simulink library "sm_car_4post_lib"  (R2021b)
settings: Solver=VariableStepAuto  StartTime=0.0  StopTime=10.0  RelTol=1e-3
values from neighbouring files (symbols this model uses):
  Init = struct    [sm_car_4post_init_data.m]
  N = 100    [sm_extr_data_cam_roller_curve.m]
  s = sin(q)    [sm_extr_data_cam_roller_curve.m]
  Vehicle = Vehicle_03    [sm_car_4post_gen_op.m]    (also in sm_car_4post_testrig_plot2testall.m)
undefined symbols (not defined in the file or in its folder): clr_upr, hp_in_f_ua, hp_in_r_ua, hp_la_out, hp_ua_out, LAc, LAf, LAr, opc_upr, radius_upr, rhs_hp, sm_car_4post_platform, smcar_param, UAc, UAf, UAr, X, Y, Z
libraries: sm_lib x234, $bdroot x71, fl_lib x24, nesl_utility x21, simulink x3
(part 1 of 11)
Description:
  | Simscape Vehicle Templates Library
settings Model: Creator=The MathWorks, Inc.  LastModifiedBy=The MathWorks, Inc.
settings SolverCC: AlgebraicLoopSolver=TrustRegion
settings DataIOCC: ReturnWorkspaceOutputs=off
settings DebuggingCC: PregeneratedLibrarySubsystemCodeDiagnostic=none  SFMachineParentedDataDiag=warning  ArithmeticOperatorsInVariantConditions=warning
settings SFSimCC: SimUseLocalCustomCode=off  CustomCodeUndefinedFunction=UseInterfaceOnly
settings RTWCC: RTWUseLocalCustomCode=off

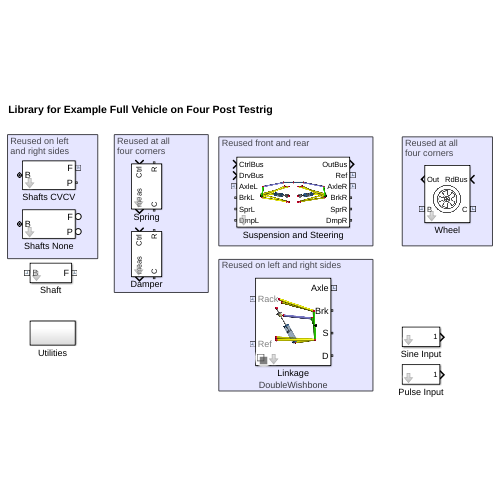
[thumbnail: Simulink's stored preview of the top-level diagram]
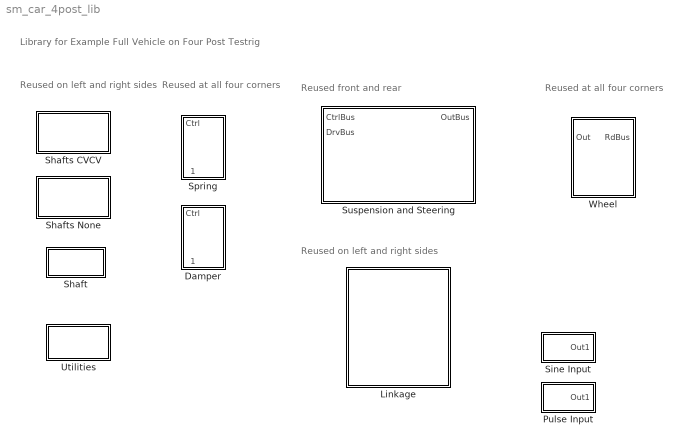
== system sm_car_4post_lib ==
  note: Reused at all
      | four corners
  note: Reused on left and right sides
  note: Reused front and rear
  note: Reused on left
      | and right sides
  note: Library for Example Full Vehicle on Four Post Testrig
  note: Reused at all
      | four corners
  Damper : Subsystem  mask(Damper){Damper=Vehicle.Chassis.Damper.Rear}
      mask prompts: Damper "Damper Parameters"
  Linkage : Subsystem  Variant=on  VariantControlMode=label  VariantControl=Variant1  LabelModeActiveChoice=DoubleWishbone  mask(Suspension){popup_leftRight=Right, Linkage=Vehicle.Chassis.SuspF.Linkage, Init=Init, VariantLabel=Vehicle.Chassis.SuspF.Linkage.class.Value, InitTriggerDropdown=1}
      mask prompts: popup_leftRight "Left/Right"; Linkage "Linkage Parameters"; Init "Initial Values"; VariantLabel "Variant Label"; InitTriggerDropdown "Initialization Trigger Dropdown"
      mask help: Suspension with multiple variants. Variants are configured by parameter Variant Label. Parameter values are contained within Linkage Parameters.
      mask init:
      | curblk = gcb;
      | 
      | % Set variant for this block 
      | set_param(curblk,'LabelModeActiveChoice',VariantLabel);
      | 
      | % Trigger Mask Initialization for 
      | % variant subsystems below this level
      | sm_car_4post_lib_maskInitTrigger(curblk)
      | 
      | % Set Left/Right fields
      | 
      | sm_car_4post_lib_setLeftRight(curblk,'variant');
      settings: AttributesFormatString=%<ActiveVariant>
      mask TypeOptions popup_leftRight: Left | Right
      mask TypeOptions InitTriggerDropdown: 0 | 1
      mask Display: image(fullfile(matlabroot,'toolbox','physmod','sm','smdemos','car_4post_testrig','images','sm_car_4post_dwbR_IMAGE.png'));
  Pulse Input : Subsystem  mask(Smooth Pulse){rise_time=0.1, pulse_length=2, wave_amplitude=5, wave_delay=1}
      mask prompts: rise_time "Rise/Fall Time (sec)"; pulse_length "Pulse Length (sec)"; wave_amplitude "Amplitude (m)"; wave_delay "Delay (sec)"
      mask help: Produces a pulse with a smooth start and finish, starting at a chosen time.
  Shaft : Subsystem  mask(Shaft){popup_leftRight=Left, shaft_m=3.5, len_shaft=0.4, clr_shaft=smcar_param.gray, opc_shaft=smcar_param.part.opc, rad_shaft=0.025}
      mask prompts: popup_leftRight "Left/Right"; shaft_m "Shaft Mass (kg)"; len_shaft "Shaft Length (m)"; clr_shaft "Color [RGB]"; opc_shaft "Opacity (0-1)"; rad_shaft "Radius (m)"
      mask help: Rigid shaft model with basic parameterization.
      mask init:
      | if(popup_leftRight == 1)
      |     rhs_shaft = 1;
      | elseif(popup_leftRight == 2)
      |     rhs_shaft = -1;
      | end
      mask TypeOptions popup_leftRight: Left | Right
      mask TypeOptions shaft_m: Shaft/Mass
      mask TypeOptions clr_shaft: Shaft/GraphicDiffuseColor
      mask TypeOptions opc_shaft: Shaft/GraphicOpacity
      mask TypeOptions rad_shaft: Shaft/CylinderRadius
      mask DialogControl cont_vis_shaft Prompt: Visualization
  Shafts CVCV : Subsystem  mask(Driveshafts){popup_leftRight=Right, Shaft=Vehicle.Driveline.ShaftsFL}
      mask prompts: popup_leftRight "Left/Right"; Shaft "Shaft Parameters"
      mask help: Driveshafts from differential to axle.
      mask init:
      | sm_car_4post_lib_setLeftRight(gcb, 'variant');
      mask TypeOptions popup_leftRight: Left | Right
  Shafts None : Subsystem  mask(Driveshaft Open Connection){popup_leftRight=Left, Shaft=Vehicle.Driveline.ShaftsRL}
      mask prompts: popup_leftRight "Left/Right"; Shaft "Shaft Parameters"
      mask help: Variant with no shaft connections, intended as a simple variant or placeholder.
      mask init:
      | sm_car_4post_lib_setLeftRight(gcb, 'variant');
      mask TypeOptions popup_leftRight: Left | Right
  Sine Input : Subsystem  mask(Sine Wave){wave_period=2, num_periods=2, wave_amplitude=5, wave_delay=1}
      mask prompts: wave_period "Period (sec)"; num_periods "Number of cycles"; wave_amplitude "Amplitude (m)"; wave_delay "Delay (sec)"
      mask help: Produces a fixed number of sine waves at a single amplitude and period, starting at a chosen time.
  Spring : Subsystem  mask(Spring){Spring=Vehicle.Chassis.Spring.Front}
      mask prompts: Spring "Spring Parameters"
  Suspension and Steering : Subsystem  mask(Suspension and Steering){Susp=Vehicle.Chassis.SuspF, Init=Init.Front, InitTriggerDropdown=0}
      mask prompts: Susp "Suspension Parameters"; Init "Initial Values"; InitTriggerDropdown "Initialization Trigger Dropdown"
      mask help: Suspension and steering system for front or rear axle.
      mask init:
      | curblk = gcb;
      | % Trigger Mask Initialization for 
      | % variant subsystems below this level
      | sm_car_4post_lib_maskInitTrigger(curblk)
      mask TypeOptions InitTriggerDropdown: 0 | 1
      mask Display: image(fullfile(matlabroot,'toolbox','physmod','sm','smdemos','car_4post_testrig','images','sm_car_4post_suspf_IMAGE.png'));
  Utilities : Subsystem
  Wheel : Subsystem  mask{popup_leftRight=Left, Tire=Vehicle.Chassis.TyreF}
      mask prompts: popup_leftRight "Left/Right"; Tire "Tire Parameters"
      mask init:
      | sm_car_4post_lib_setLeftRight(gcb,'variant');
      mask TypeOptions popup_leftRight: Left | Right
      mask Display: image(fullfile(matlabroot,'toolbox','physmod','sm','smdemos','car_4post_testrig','images','sm_car_4post_wheel_IMAGE.png'));

== system sm_car_4post_lib/Damper ==
  Ctrl : Inport
  Linear : Subsystem  VariantControl=Linear  mask(Linear Damper with Hard Stop){dam_b=Damper.Damping.d.Value, hp_dpr_top=Damper.Damping.sTop.Value, hp_dpr_bot=Damper.Damping.sBottom.Value, bs_lim_upper=Damper.Endstop.xMax.Value, bs_lim_lower=Damper.Endstop.xMin.Value, bs_k_upper=Damper.Endstop.KxMax.Value, bs_k_lower=Damper.Endstop.KxMin.Value, bs_b_upper=Damper.Endstop.dxMax.Value, bs_b_lower=Damper.Endstop.dxMin.Value, bs_region=Damper.Endstop.xTransition.Value}
      mask prompts: dam_b "Damper (N/(m/s))"; hp_dpr_top "HP Damper Top [xyz] (m)"; hp_dpr_bot "HP Damper Bottom [xyz] (m)"; bs_region "Transition Region (m)"
      mask help: Damper and hard stop with linear behavior with measurements.
      mask init:
      | dam_x0 = norm(hp_dpr_top - hp_dpr_bot);
      mask TypeOptions dam_b: Damper/D
      mask DialogControl text_bumpstop_upper Prompt: Upper
      mask DialogControl text_bumpstop_lower Prompt: Lower
      mask DialogControl text_bumpstop_limit Prompt: Limit (m)
      mask DialogControl text_bumpstop_k Prompt: Stiffness (N/m)
      mask DialogControl text_bumpstop_b Prompt: Damping  (N/(m/s))
  R : PMIOPort  Side=Left
  C : PMIOPort  Port=2  Side=Right
  meas : Outport  VectorParamsAs1DForOutWhenUnconnected=off
  wires:
  Linear/1(meas) -> meas/1
  Ctrl/1 -> Linear/1(Ctrl)
  connections:
  Linear/LConn1 -- R/RConn1
  Linear/RConn1 -- C/RConn1

== system sm_car_4post_lib/Linkage ==
  DoubleWishbone : Subsystem  VariantControl=DoubleWishbone  mask(Double-Wishbone Suspension){popup_leftRight=Right, hp_in_f_ua=Linkage.UpperWishbone.sInboardF.Value, hp_in_r_ua=Linkage.UpperWishbone.sInboardR.Value, hp_out_ua=Linkage.UpperWishbone.sOutboard.Value, hp_in_f_la=Linkage.LowerWishbone.sInboardF.Value, hp_in_r_la=Linkage.LowerWishbone.sInboardR.Value, hp_out_la=Linkage.LowerWishbone.sOutboard.Value, hp_upr_cg=Linkage.Upright.sCG.Value, hp_upr_wc=Linkage.Upright.sWheelCentre.Value, hp_in_rod=Linkage.TrackRod.sInboard.Value, hp_upr_rod=Linkage.TrackRod.sOutboard.Value, hp_spr_top=Linkage.Shock.sTop.Value, hp_spr_bot=Linkage.Shock.sBottom.Value, clr_hp=smcar_param.hp.clr, opc_hp=smcar_param.hp.opc, size_hp=0.025, ua_mass=Linkage.UpperWishbone.m.Value, clr_ua=smcar_param.yellow, opc_ua=smcar_param.part.opc, radius_ua=0.02, la_mass=Linkage.LowerWishbone.m.Value, clr_la=smcar_param.yellow, opc_la=smcar_param.part.opc, radius_la=0.02, shock_pist_mass=Linkage.Shock.mPiston.Value, shock_cyl_mass=Linkage.Shock.mCylinder.Value, up_lim_bumpstop=Linkage.Endstop.xMax.Value, low_lim_bumpstop=Linkage.Endstop.xMin.Value, clr_conn_shock=smcar_param.hp.clr, opc_conn_shock=smcar_param.hp.opc, size_conn_shock=0.025, clr_shock_cyl=smcar_param.blue, opc_shock_cyl=1.0, radius_shock_cyl=0.05, clr_shock_piston=smcar_param.gray, opc_shock_piston=1.0, clr_shock_bumpstop=smcar_param.yellowpale, opc_shock_bumpstop=1.0, deadvol_len_shock_cyl=smcar_param.shock.dead_length, piston_len_shock=smcar_param.shock.piston, cyl_cap_len_shock=smcar_param.shock.cap, bumpstop_len_shock=smcar_param.shock.bumpstop_len, upr_mass=Linkage.Upright.m.Value, atoe=Linkage.Upright.aToe.Value, acamber=Linkage.Upright.aCamber.Value, clr_conn_upr=smcar_param.hp.clr, opc_conn_upr=smcar_param.hp.opc, size_conn_upr=smcar_param.hp.rad, clr_upr=smcar_param.green, opc_upr=smcar_param.part.opc, radius_upr=0.02, clr_stub_axle=smcar_param.black, opc_stub_axle=smcar_param.part.opc, radius_stub_axle=0.02, rod_mass=Linkage.TrackRod.m.Value, clr_conn_rod=smcar_param.hp.clr, opc_conn_rod=smcar_param.hp.opc, size_conn_rod=smcar_param.hp.rad, clr_rod=smcar_param.purple, opc_rod=smcar_param.part.opc, radius_rod=0.02, whl_init_spd_lr=Init.nWheel.Value, whlind=1}
      mask prompts: popup_leftRight "Left/Right"; hp_in_f_ua "Upper Arm Front [xyz] (m)"; hp_in_r_ua "Upper Arm Rear [xyz] (m)"; hp_out_ua "Upper Arm Outboard [xyz] (m)"; hp_in_f_la "Lower Arm Front [xyz] (m)"; hp_in_r_la "Lower Arm Rear [xyz] (m)"; hp_out_la "Lower Arm Outboard [xyz] (m)"; hp_upr_cg "Upright CG [xyz] (m)"; hp_upr_wc "Wheel Center [xyz] (m)"; hp_in_rod "Track Rod Inboard [xyz] (m)"; hp_upr_rod "Track Rod Outboard [xyz] (m)"; hp_spr_top "Spring Top [xyz] (m)"; hp_spr_bot "Spring Bottom [xyz] (m)"; ua_mass "Mass (kg)"; clr_ua "Color [RGB]"; opc_ua "Opacity (0-1)"; radius_ua "Radius (m)"; la_mass "Mass (kg)"; clr_la "Color [RGB]"; opc_la "Opacity (0-1)"; radius_la "Radius (m)"; shock_pist_mass "Piston Mass (kg)"; shock_cyl_mass "Cylinder Mass (kg)"; up_lim_bumpstop "Upper Limit (m)"; low_lim_bumpstop "Lower Limit (m)"; deadvol_len_shock_cyl "Dead Volume Height (m)"; piston_len_shock "Piston Length (m)"; cyl_cap_len_shock "Cylinder Cap Length (m)"; bumpstop_len_shock "Bumpstop Length (m)"; upr_mass "Mass (kg)"; atoe "Toe Angle (deg)"; acamber "Camber Angle (deg)"; rod_mass "Mass (kg)"; whl_init_spd_lr "Initial Wheel Speed (rad/s)"; whlind "Wheel Index"
      mask help: This models a double-wishbone suspension for steered and non-steered configurations. The non-steered configuration maintains its orientation via the track rods that connect to fixed points on the subframe.
      mask init:
      | sm_car_4post_lib_setLeftRight(gcb,'none');
      | 
      | if(popup_leftRight == 1)
      |     rhs_susp = 1;
      |     whlind = 1;
      | elseif(popup_leftRight == 2)
      |     rhs_susp = -1;
      |     whlind = 2;
      | end
      mask TypeOptions popup_leftRight: Left | Right
      mask TypeOptions hp_in_f_ua: Upper Arm/hp_in_f | Hardpoints/hp_in_f_ua
      mask TypeOptions hp_in_r_ua: Upper Arm/hp_in_r | Hardpoints/hp_in_r_ua
      mask TypeOptions hp_out_ua: Upper Arm/hp_out | Upright/hp_ua_out
      mask TypeOptions hp_in_f_la: Lower Arm/hp_in_f | Hardpoints/hp_in_f_la
      mask TypeOptions hp_in_r_la: Lower Arm/hp_in_r | Hardpoints/hp_in_r_la
      mask TypeOptions hp_out_la: Lower Arm/hp_out | Upright/hp_la_out
      mask TypeOptions hp_upr_cg: Upright/hp_upr_cg
      mask TypeOptions hp_upr_wc: Upright/hp_upr_wc
      mask TypeOptions hp_in_rod: Track Rod/hp_in
      mask TypeOptions hp_upr_rod: Track Rod/hp_out | Upright/hp_upr_rod
      mask TypeOptions hp_spr_top: Hardpoints/hp_spr_top | Shock/hp_spr_top
      mask TypeOptions hp_spr_bot: Lower Arm/hp_spr | Shock/hp_spr_bot
      mask TypeOptions clr_hp: Hardpoints/clr_hp
      mask TypeOptions opc_hp: Hardpoints/opc_hp
      mask TypeOptions size_hp: Hardpoints/size_hp
      mask TypeOptions ua_mass: Upper Arm/ua_mass
      mask TypeOptions clr_ua: Upper Arm/clr_ua
      mask TypeOptions opc_ua: Upper Arm/opc_ua
      mask TypeOptions radius_ua: Upper Arm/radius_ua
      mask TypeOptions la_mass: Lower Arm/la_mass
      mask TypeOptions clr_la: Lower Arm/clr_la
      mask TypeOptions opc_la: Lower Arm/opc_la
      mask TypeOptions radius_la: Lower Arm/radius_la
      mask TypeOptions shock_pist_mass: Shock/shock_pist_mass
      mask TypeOptions shock_cyl_mass: Shock/shock_cyl_mass
      mask TypeOptions up_lim_bumpstop: Shock/up_lim_bumpstop
      mask TypeOptions low_lim_bumpstop: Shock/low_lim_bumpstop
      mask TypeOptions clr_conn_shock: Shock/clr_conn_shock
      mask TypeOptions opc_conn_shock: Shock/opc_conn_shock
      mask TypeOptions size_conn_shock: Shock/size_conn_shock
      mask TypeOptions clr_shock_cyl: Shock/clr_shock_cyl
      mask TypeOptions opc_shock_cyl: Shock/opc_shock_cyl
      mask TypeOptions radius_shock_cyl: Shock/radius_shock_cyl
      mask TypeOptions clr_shock_piston: Shock/clr_shock_piston
      mask TypeOptions opc_shock_piston: Shock/opc_shock_piston
      mask TypeOptions clr_shock_bumpstop: Shock/clr_shock_bumpstop
      mask TypeOptions opc_shock_bumpstop: Shock/opc_shock_bumpstop
      mask TypeOptions deadvol_len_shock_cyl: Shock/deadvol_len_shock_cyl
      mask TypeOptions piston_len_shock: Shock/piston_len_shock
      mask TypeOptions cyl_cap_len_shock: Shock/cyl_cap_len_shock
      mask TypeOptions bumpstop_len_shock: Shock/bumpstop_len_shock
      mask TypeOptions upr_mass: Upright/upr_mass
      mask TypeOptions atoe: Upright/atoe
      mask TypeOptions acamber: Upright/acamber
      mask TypeOptions clr_conn_upr: Upright/clr_conn_upr
      mask TypeOptions opc_conn_upr: Upright/opc_conn_upr
      mask TypeOptions size_conn_upr: Upright/size_conn_upr
      mask TypeOptions clr_upr: Upright/clr_upr
      mask TypeOptions opc_upr: Upright/opc_upr
      mask TypeOptions radius_upr: Upright/radius_upr
      mask TypeOptions clr_stub_axle: Upright/clr_stub_axle
      mask TypeOptions opc_stub_axle: Upright/opc_stub_axle
      mask TypeOptions radius_stub_axle: Upright/radius_stub_axle
      mask TypeOptions rod_mass: Track Rod/rod_mass
      mask TypeOptions clr_conn_rod: Track Rod/clr_conn_rod
      mask TypeOptions opc_conn_rod: Track Rod/opc_conn_rod
      mask TypeOptions size_conn_rod: Track Rod/size_conn_rod
      mask TypeOptions clr_rod: Track Rod/clr_rod
      mask TypeOptions opc_rod: Track Rod/opc_rod
      mask TypeOptions radius_rod: Track Rod/radius_rod
      mask DialogControl cont_hp Prompt: Hardpoints
      mask DialogControl cont_vis_hp Prompt: Visualization
      mask DialogControl text_clr_hp Prompt: Color [RGB]
      mask DialogControl text_opc_hp Prompt: Opac. (0-1)
      mask DialogControl text_size_hp Prompt: Size (m)
      mask DialogControl text_hp Prompt: Hardpoints
      mask DialogControl cont_ua Prompt: UA
      mask DialogControl cont_vis_ua Prompt: Visualization
      mask DialogControl cont_la Prompt: LA
      mask DialogControl cont_vis_la Prompt: Visualization
      mask DialogControl cont_shock Prompt: Shock
      mask DialogControl cont_parts Prompt: Parts
      mask DialogControl cont_bumpstop Prompt: Bumpstop
      mask DialogControl cont_vis_shock Prompt: Visualization
      mask DialogControl text_clr_shock Prompt: Color  [RGB]
      mask DialogControl text_opc_shock Prompt: Opac. (0-1)
      mask DialogControl text_size_shock Prompt: Size (m)
      mask DialogControl text_conn_shock Prompt: Connections
      mask DialogControl text_shock_shock Prompt: Cylinder
      mask DialogControl text_shock_piston Prompt: Piston
      mask DialogControl text_piston_radius Prompt: <cylinder radius>
      mask DialogControl text_shock_bumpstop Prompt: Bumpstop
      mask DialogControl text_bumpstop_radius Prompt: <cylinder radius>
      mask DialogControl cont_upright Prompt: Upright
      mask DialogControl grp_upright Prompt: Upright
      mask DialogControl cont_vis_upr Prompt: Visualization
      mask DialogControl text_clr_upr Prompt: Color [RGB]
      mask DialogControl text_opc_upr Prompt: Opac. (0-1)
      mask DialogControl text_size_upr Prompt: Size (m)
      mask DialogControl text_conn_upr Prompt: Connections
      mask DialogControl text_upright Prompt: Upright
      mask DialogControl text_stub_axle Prompt: Stub Axle
      mask DialogControl cont_steer Prompt: Steer
      mask DialogControl grp_rod Prompt: Rod
      mask DialogControl cont_vis_rod Prompt: Visualization
      mask DialogControl text_clr_rod Prompt: Color [RGB]
      mask DialogControl text_opc_rod Prompt: Opac. (0-1)
      mask DialogControl text_size_rod Prompt: Size (m)
      mask DialogControl text_conn_rod Prompt: Connections
      mask DialogControl text_rod_rod Prompt: Rod
      mask DialogControl cont_init Prompt: Initial
      mask Display: image(fullfile(matlabroot,'toolbox','physmod','sm','smdemos','car_4post_testrig','images','sm_car_4post_dwbR_IMAGE.png'));
  FiveLinkShockRear : Subsystem  VariantControl=FiveLinkShockRear  mask(Five-Link Suspension, Shock to Rear){popup_leftRight=Right, hp_in_f_ua=Linkage.UpperArmF.sInboard.Value, hp_in_r_ua=Linkage.UpperArmR.sInboard.Value, hp_out_f_ua=Linkage.UpperArmF.sOutboard.Value, hp_out_r_ua=Linkage.UpperArmR.sOutboard.Value, hp_in_f_la=Linkage.LowerArmF.sInboard.Value, hp_in_r_la=Linkage.LowerArmR.sInboard.Value, hp_out_f_la=Linkage.LowerArmF.sOutboard.Value, hp_out_r_la=Linkage.LowerArmR.sOutboard.Value, hp_upr_cg=Linkage.Upright.sCG.Value, hp_upr_wc=Linkage.Upright.sWheelCentre.Value, hp_in_rod=Linkage.TrackRod.sInboard.Value, hp_upr_rod=Linkage.TrackRod.sOutboard.Value, hp_spr_top=Linkage.Shock.sTop.Value, hp_spr_bot=Linkage.Shock.sBottom.Value, clr_hp=smcar_param.hp.clr, opc_hp=smcar_param.hp.opc, size_hp=0.025, uaf_mass=Linkage.UpperArmF.m.Value, uar_mass=Linkage.UpperArmR.m.Value, laf_mass=Linkage.LowerArmF.m.Value, lar_mass=Linkage.LowerArmR.m.Value, clr_conn_links=smcar_param.hp.clr, opc_conn_links=smcar_param.hp.opc, size_conn_links=smcar_param.hp.rad, clr_uaf=smcar_param.yellow, opc_uaf=smcar_param.part.opc, radius_uaf=0.02, clr_uar=smcar_param.yellow, opc_uar=smcar_param.part.opc, radius_uar=0.02, clr_laf=smcar_param.yellow, opc_laf=smcar_param.part.opc, radius_laf=0.02, clr_lar=smcar_param.yellow, opc_lar=smcar_param.part.opc, radius_lar=0.02, shock_pist_mass=Linkage.Shock.mPiston.Value, shock_cyl_mass=Linkage.Shock.mCylinder.Value, up_lim_bumpstop=Linkage.Endstop.xMax.Value, low_lim_bumpstop=Linkage.Endstop.xMin.Value, clr_conn_shock=smcar_param.hp.clr, opc_conn_shock=smcar_param.hp.opc, size_conn_shock=0.025, clr_shock_cyl=smcar_param.blue, opc_shock_cyl=1.0, radius_shock_cyl=0.05, clr_shock_piston=smcar_param.gray, opc_shock_piston=1.0, clr_shock_bumpstop=smcar_param.yellowpale, opc_shock_bumpstop=1.0, deadvol_len_shock_cyl=smcar_param.shock.dead_length, piston_len_shock=smcar_param.shock.piston, cyl_cap_len_shock=smcar_param.shock.cap, bumpstop_len_shock=smcar_param.shock.bumpstop_len, atoe=Linkage.Upright.aToe.Value, acamber=Linkage.Upright.aCamber.Value, upr_mass=Linkage.Upright.m.Value, clr_conn_upr=smcar_param.hp.clr, opc_conn_upr=smcar_param.hp.opc, size_conn_upr=smcar_param.hp.rad, clr_upr=smcar_param.green, opc_upr=smcar_param.part.opc, radius_upr=0.02, clr_stub_axle=smcar_param.black, opc_stub_axle=smcar_param.part.opc, radius_stub_axle=0.02, rod_mass=Linkage.TrackRod.m.Value, clr_conn_rod=smcar_param.hp.clr, opc_conn_rod=smcar_param.hp.opc, size_conn_rod=smcar_param.hp.rad, clr_rod=smcar_param.purple, opc_rod=smcar_param.part.opc, radius_rod=0.02, whl_init_spd_lr=Init.nWheel.Value}
      mask prompts: popup_leftRight "Left/Right"; hp_in_f_ua "Upper Arm Front [xyz] (m)"; hp_in_r_ua "Upper Arm Rear [xyz] (m)"; hp_out_f_ua "Upper Arm Front Outboard [xyz] (m)"; hp_out_r_ua "Upper Arm Rear Outboard [xyz] (m)"; hp_in_f_la "Lower Arm Front [xyz] (m)"; hp_in_r_la "Lower Arm Rear [xyz] (m)"; hp_out_f_la "Lower Arm Front Outboard [xyz] (m)"; hp_out_r_la "Lower Arm Rear Outboard [xyz] (m)"; hp_upr_cg "Upright CG [xyz] (m)"; hp_upr_wc "Wheel Center [xyz] (m)"; hp_in_rod "Track Rod Inboard [xyz] (m)"; hp_upr_rod "Track Rod Outboard [xyz] (m)"; hp_spr_top "Spring Top [xyz] (m)"; hp_spr_bot "Spring Bottom [xyz] (m)"; shock_pist_mass "Piston Mass (kg)"; shock_cyl_mass "Cylinder Mass (kg)"; up_lim_bumpstop "Upper Limit (m)"; low_lim_bumpstop "Lower Limit (m)"; deadvol_len_shock_cyl "Dead Volume Height (m)"; piston_len_shock "Piston Length (m)"; cyl_cap_len_shock "Cylinder Cap Length (m)"; bumpstop_len_shock "Bumpstop Length (m)"; atoe "Toe Angle (deg)"; acamber "Camber Angle (deg)"; upr_mass "Mass (kg)"; rod_mass "Mass (kg)"; whl_init_spd_lr "Initial Wheel Speed (rad/s)"
      mask help: Models a multi-link suspension with two upper and two lower control arms connecting the subframe to the upright. The shock is connected to the subframe and rear lower arm link.
      mask init:
      | sm_car_4post_lib_setLeftRight(gcb,'none');
      | 
      | if(popup_leftRight == 1)
      |     rhs_susp = 1;
      |     whlind = 1;
      | elseif(popup_leftRight == 2)
      |     rhs_susp = -1;
      |     whlind = 2;
      | end
      mask TypeOptions popup_leftRight: Left | Right
      mask TypeOptions hp_in_f_ua:
      | Hardpoints/hp_in_f_ua | Upper Arm Front/hp_in | Universal
      | HP UAF/hp_f | Universal
      | HP UAR/hp_f
      mask TypeOptions hp_in_r_ua:
      | Hardpoints/hp_in_r_ua | Upper Arm Rear/hp_in | Universal
      | HP UAF/hp_r | Universal
      | HP UAR/hp_r
      mask TypeOptions hp_out_f_ua: Upper Arm Front/hp_out | Upright/hp_uaf_out
      mask TypeOptions hp_out_r_ua: Upper Arm Rear/hp_out | Upright/hp_uar_out
      mask TypeOptions hp_in_f_la:
      | Hardpoints/hp_in_f_la | Lower Arm Front/hp_in | Universal
      | HP LAF/hp_f | Universal
      | HP LAR/hp_f
      mask TypeOptions hp_in_r_la:
      | Hardpoints/hp_in_r_la | Lower Arm Rear/hp_in | Universal
      | HP LAF/hp_r | Universal
      | HP LAR/hp_r
      mask TypeOptions hp_out_f_la: Upright/hp_laf_out | Lower Arm Front/hp_out
      mask TypeOptions hp_out_r_la: Upright/hp_lar_out | Lower Arm Rear/hp_out
      mask TypeOptions hp_upr_cg: Upright/hp_upr_cg
      mask TypeOptions hp_upr_wc: Upright/hp_upr_wc
      mask TypeOptions hp_in_rod: Track Rod/hp_in
      mask TypeOptions hp_upr_rod: Track Rod/hp_out | Upright/hp_upr_rod
      mask TypeOptions hp_spr_top: Hardpoints/hp_spr_top | Shock Absorber/hp_spr_top
      mask TypeOptions hp_spr_bot: Shock Absorber/hp_spr_bot | Lower Arm Rear/hp_spr
      mask TypeOptions clr_hp: Hardpoints/clr_hp
      mask TypeOptions opc_hp: Hardpoints/opc_hp
      mask TypeOptions size_hp: Hardpoints/size_hp
      mask TypeOptions uaf_mass: Upper Arm Front/rod_mass
      mask TypeOptions uar_mass: Upper Arm Rear/rod_mass
      mask TypeOptions laf_mass: Lower Arm Front/rod_mass
      mask TypeOptions lar_mass: Lower Arm Rear/rod_mass
      mask TypeOptions clr_conn_links: Upper Arm Front/clr_conn_rod | Upper Arm Rear/clr_conn_rod | Lower Arm Front/clr_conn_rod | Lower Arm Rear/clr_conn_rod
      mask TypeOptions opc_conn_links: Upper Arm Front/opc_conn_rod | Upper Arm Rear/opc_conn_rod | Lower Arm Front/opc_conn_rod | Lower Arm Rear/opc_conn_rod
      mask TypeOptions size_conn_links: Upper Arm Front/size_conn_rod | Upper Arm Rear/size_conn_rod | Lower Arm Front/size_conn_rod | Lower Arm Rear/size_conn_rod
      mask TypeOptions clr_uaf: Upper Arm Front/clr_rod
      mask TypeOptions opc_uaf: Upper Arm Front/opc_rod
      mask TypeOptions radius_uaf: Upper Arm Front/radius_rod
      mask TypeOptions clr_uar: Upper Arm Rear/clr_rod
      mask TypeOptions opc_uar: Upper Arm Rear/opc_rod
      mask TypeOptions radius_uar: Upper Arm Rear/radius_rod
      mask TypeOptions clr_laf: Lower Arm Front/clr_rod
      mask TypeOptions opc_laf: Lower Arm Front/opc_rod
      mask TypeOptions radius_laf: Lower Arm Front/radius_rod
      mask TypeOptions clr_lar: Lower Arm Rear/clr_rod
      mask TypeOptions opc_lar: Lower Arm Rear/opc_rod
      mask TypeOptions radius_lar: Lower Arm Rear/radius_rod
      mask TypeOptions shock_pist_mass: Shock Absorber/shock_pist_mass
      mask TypeOptions shock_cyl_mass: Shock Absorber/shock_cyl_mass
      mask TypeOptions up_lim_bumpstop: Shock Absorber/up_lim_bumpstop
      mask TypeOptions low_lim_bumpstop: Shock Absorber/low_lim_bumpstop
      mask TypeOptions clr_conn_shock: Shock Absorber/clr_conn_shock
      mask TypeOptions opc_conn_shock: Shock Absorber/opc_conn_shock
      mask TypeOptions size_conn_shock: Shock Absorber/size_conn_shock
      mask TypeOptions clr_shock_cyl: Shock Absorber/clr_shock_cyl
      mask TypeOptions opc_shock_cyl: Shock Absorber/opc_shock_cyl
      mask TypeOptions radius_shock_cyl: Shock Absorber/radius_shock_cyl
      mask TypeOptions clr_shock_piston: Shock Absorber/clr_shock_piston
      mask TypeOptions opc_shock_piston: Shock Absorber/opc_shock_piston
      mask TypeOptions clr_shock_bumpstop: Shock Absorber/clr_shock_bumpstop
      mask TypeOptions opc_shock_bumpstop: Shock Absorber/opc_shock_bumpstop
      mask TypeOptions deadvol_len_shock_cyl: Shock Absorber/deadvol_len_shock_cyl
      mask TypeOptions piston_len_shock: Shock Absorber/piston_len_shock
      mask TypeOptions cyl_cap_len_shock: Shock Absorber/cyl_cap_len_shock
      mask TypeOptions bumpstop_len_shock: Shock Absorber/bumpstop_len_shock
      mask TypeOptions atoe: Upright/atoe
      mask TypeOptions acamber: Upright/acamber
      mask TypeOptions upr_mass: Upright/upr_mass
      mask TypeOptions clr_conn_upr: Upright/clr_conn_upr
      mask TypeOptions opc_conn_upr: Upright/opc_conn_upr
      mask TypeOptions size_conn_upr: Upright/size_conn_upr
      mask TypeOptions clr_upr: Upright/clr_upr
      mask TypeOptions opc_upr: Upright/opc_upr
      mask TypeOptions radius_upr: Upright/radius_upr
      mask TypeOptions clr_stub_axle: Upright/clr_stub_axle
      mask TypeOptions opc_stub_axle: Upright/opc_stub_axle
      mask TypeOptions radius_stub_axle: Upright/radius_stub_axle
      mask TypeOptions rod_mass: Track Rod/rod_mass
      mask TypeOptions clr_conn_rod: Track Rod/clr_conn_rod
      mask TypeOptions opc_conn_rod: Track Rod/opc_conn_rod
      mask TypeOptions size_conn_rod: Track Rod/size_conn_rod
      mask TypeOptions clr_rod: Track Rod/clr_rod
      mask TypeOptions opc_rod: Track Rod/opc_rod
      mask TypeOptions radius_rod: Track Rod/radius_rod
      mask DialogControl cont_hp Prompt: Hardpoints
      mask DialogControl cont_vis_hp Prompt: Visualization
      mask DialogControl text_clr_hp Prompt: Color [RGB]
      mask DialogControl text_opc_hp Prompt: Opac. (0-1)
      mask DialogControl text_size_hp Prompt: Size (m)
      mask DialogControl text_hp Prompt: Hardpoints
      mask DialogControl cont_links Prompt: Links
      mask DialogControl text_links_part Prompt: Part
      mask DialogControl text_links_mass Prompt: Mass (kg)
      mask DialogControl text_upper_f Prompt: Upper, Front
      mask DialogControl text_upper_r Prompt: Upper, Rear
      mask DialogControl text_lower_f Prompt: Lower, Front
      mask DialogControl text_lower_r Prompt: Lower, Rear
      mask DialogControl cont_vis_links Prompt: Visualization
      mask DialogControl text_vis_links_clr Prompt: Color [RGB]
      mask DialogControl text_vis_links_opc Prompt: Opacity (0-1)
      mask DialogControl text_vis_links_rad Prompt: Radius (m)
      mask DialogControl text_vis_links_conn Prompt: Connections
      mask DialogControl text_vis_links_uaf Prompt: Upper, Front
      mask DialogControl text_vis_links_uar Prompt: Upper, Rear
      mask DialogControl text_vis_links_laf Prompt: Lower, Front
      mask DialogControl text_vis_links_lar Prompt: Lower, Rear
      mask DialogControl cont_shock Prompt: Shock
      mask DialogControl cont_parts Prompt: Parts
      mask DialogControl cont_bumpstop Prompt: Bumpstop
      mask DialogControl cont_vis_shock Prompt: Visualization
      mask DialogControl text_clr_shock Prompt: Color  [RGB]
      mask DialogControl text_opc_shock Prompt: Opac. (0-1)
      mask DialogControl text_size_shock Prompt: Size (m)
      mask DialogControl text_conn_shock Prompt: Connections
      mask DialogControl text_shock_shock Prompt: Cylinder
      mask DialogControl text_shock_piston Prompt: Piston
      mask DialogControl text_piston_radius Prompt: <cylinder radius>
      mask DialogControl text_shock_bumpstop Prompt: Bumpstop
      mask DialogControl text_bumpstop_radius Prompt: <cylinder radius>
      mask DialogControl cont_upright Prompt: Upright
      mask DialogControl grp_upright Prompt: Upright
      mask DialogControl cont_vis_upr Prompt: Visualization
      mask DialogControl text_clr_upr Prompt: Color [RGB]
      mask DialogControl text_opc_upr Prompt: Opac. (0-1)
      mask DialogControl text_size_upr Prompt: Size (m)
      mask DialogControl text_conn_upr Prompt: Connections
      mask DialogControl text_upright Prompt: Upright
      mask DialogControl text_stub_axle Prompt: Stub Axle
      mask DialogControl cont_steer Prompt: Steer
      mask DialogControl grp_rod Prompt: Rod
      mask DialogControl cont_vis_rod Prompt: Visualization
      mask DialogControl text_clr_rod Prompt: Color [RGB]
      mask DialogControl text_opc_rod Prompt: Opac. (0-1)
      mask DialogControl text_size_rod Prompt: Size (m)
      mask DialogControl text_conn_rod Prompt: Connections
      mask DialogControl text_rod_rod Prompt: Rod
      mask DialogControl cont_initial Prompt: Initial
      mask Display: image(fullfile(matlabroot,'toolbox','physmod','sm','smdemos','car_4post_testrig','images','sm_car_4post_dwbR_IMAGE.png'));
  SplitLowerArmShockFront : Subsystem  VariantControl=SplitLowerArmShockFront  mask(Split Lower Arm, Shock to Front Lower Arm){popup_leftRight=Right, hp_in_f_ua=Linkage.UpperWishbone.sInboardF.Value, hp_in_r_ua=Linkage.UpperWishbone.sInboardR.Value, hp_out_ua=Linkage.UpperWishbone.sOutboard.Value, hp_in_f_la=Linkage.LowerArmF.sInboard.Value, hp_in_r_la=Linkage.LowerArmR.sInboard.Value, hp_out_f_la=Linkage.LowerArmF.sOutboard.Value, hp_out_r_la=Linkage.LowerArmR.sOutboard.Value, hp_upr_cg=Linkage.Upright.sCG.Value, hp_upr_wc=Linkage.Upright.sWheelCentre.Value, hp_in_rod=Linkage.TrackRod.sInboard.Value, hp_upr_rod=Linkage.TrackRod.sOutboard.Value, hp_spr_top=Linkage.Shock.sTop.Value, hp_spr_bot=Linkage.Shock.sBottom.Value, clr_hp=smcar_param.hp.clr, opc_hp=smcar_param.hp.opc, size_hp=0.025, ua_mass=Linkage.UpperWishbone.m.Value, clr_ua=smcar_param.yellow, opc_ua=smcar_param.part.opc, radius_ua=0.02, laf_mass=Linkage.LowerArmF.m.Value, lar_mass=Linkage.LowerArmR.m.Value, clr_conn_la=smcar_param.hp.clr, opc_conn_la=smcar_param.hp.opc, size_conn_la=smcar_param.hp.rad, clr_laf=smcar_param.yellow, opc_laf=smcar_param.part.opc, radius_laf=0.02, clr_lar=smcar_param.yellow, opc_lar=smcar_param.part.opc, radius_lar=0.02, shock_pist_mass=Linkage.Shock.mPiston.Value, shock_cyl_mass=Linkage.Shock.mCylinder.Value, up_lim_bumpstop=Linkage.Endstop.xMax.Value, low_lim_bumpstop=Linkage.Endstop.xMin.Value, clr_conn_shock=smcar_param.hp.clr, opc_conn_shock=smcar_param.hp.opc, size_conn_shock=0.025, clr_shock_cyl=smcar_param.blue, opc_shock_cyl=1.0, radius_shock_cyl=0.05, clr_shock_piston=smcar_param.gray, opc_shock_piston=1.0, clr_shock_bumpstop=smcar_param.yellowpale, opc_shock_bumpstop=1.0, deadvol_len_shock_cyl=smcar_param.shock.dead_length, piston_len_shock=smcar_param.shock.piston, cyl_cap_len_shock=smcar_param.shock.cap, bumpstop_len_shock=smcar_param.shock.bumpstop_len, atoe=Linkage.Upright.aToe.Value, acamber=Linkage.Upright.aCamber.Value, upr_mass=Linkage.Upright.m.Value, clr_conn_upr=smcar_param.hp.clr, opc_conn_upr=smcar_param.hp.opc, size_conn_upr=smcar_param.hp.rad, clr_upr=smcar_param.green, opc_upr=smcar_param.part.opc, radius_upr=0.02, clr_stub_axle=smcar_param.black, opc_stub_axle=smcar_param.part.opc, radius_stub_axle=0.02, rod_mass=Linkage.TrackRod.m.Value, clr_conn_rod=smcar_param.hp.clr, opc_conn_rod=smcar_param.hp.opc, size_conn_rod=smcar_param.hp.rad, clr_rod=smcar_param.purple, opc_rod=smcar_param.part.opc, radius_rod=0.02, whl_init_spd_lr=Init.nWheel.Value}
      mask prompts: popup_leftRight "Left/Right"; hp_in_f_ua "Upper Arm Front [xyz] (m)"; hp_in_r_ua "Upper Arm Rear [xyz] (m)"; hp_out_ua "Upper Arm Outboard [xyz] (m)"; hp_in_f_la "Lower Arm Front [xyz] (m)"; hp_in_r_la "Lower Arm Rear [xyz] (m)"; hp_out_f_la "Lower Arm Front Outboard [xyz] (m)"; hp_out_r_la "Lower Arm Rear Outboard [xyz] (m)"; hp_upr_cg "Upright CG [xyz] (m)"; hp_upr_wc "Wheel Center [xyz] (m)"; hp_in_rod "Track Rod Inboard [xyz] (m)"; hp_upr_rod "Track Rod Outboard [xyz] (m)"; hp_spr_top "Spring Top [xyz] (m)"; hp_spr_bot "Spring Bottom [xyz] (m)"; ua_mass "Mass (kg)"; clr_ua "Color [RGB]"; opc_ua "Opacity (0-1)"; radius_ua "Radius (m)"; shock_pist_mass "Piston Mass (kg)"; shock_cyl_mass "Cylinder Mass (kg)"; up_lim_bumpstop "Upper Limit (m)"; low_lim_bumpstop "Lower Limit (m)"; deadvol_len_shock_cyl "Dead Volume Height (m)"; piston_len_shock "Piston Length (m)"; cyl_cap_len_shock "Cylinder Cap Length (m)"; bumpstop_len_shock "Bumpstop Length (m)"; atoe "Toe Angle (deg)"; acamber "Camber Angle (deg)"; upr_mass "Mass (kg)"; rod_mass "Mass (kg)"; whl_init_spd_lr "Initial Wheel Speed (rad/s)"
      mask help: Models a suspension with upper wishbone, lower arm as two separate links connected to the upright. The shock is connected to the subframe and front lower arm link.
      mask init:
      | sm_car_4post_lib_setLeftRight(gcb,'none');
      | 
      | if(popup_leftRight == 1)
      |     rhs_susp = 1;
      |     whlind = 1;
      | elseif(popup_leftRight == 2)
      |     rhs_susp = -1;
      |     whlind = 2;
      | end
      mask TypeOptions popup_leftRight: Left | Right
      mask TypeOptions hp_in_f_ua: Upper Arm/hp_in_f | Hardpoints/hp_in_f_ua
      mask TypeOptions hp_in_r_ua: Upper Arm/hp_in_r | Hardpoints/hp_in_r_ua
      mask TypeOptions hp_out_ua: Upper Arm/hp_out | Upright/hp_ua_out
      mask TypeOptions hp_in_f_la:
      | Hardpoints/hp_in_f_la | Lower Arm Front/hp_in | Universal
      | HP LAF/hp_f | Universal
      | HP LAR/hp_f
      mask TypeOptions hp_in_r_la:
      | Hardpoints/hp_in_r_la | Lower Arm Rear/hp_in | Universal
      | HP LAF/hp_r | Universal
      | HP LAR/hp_r
      mask TypeOptions hp_out_f_la: Upright/hp_laf_out | Lower Arm Front/hp_out
      mask TypeOptions hp_out_r_la: Upright/hp_lar_out | Lower Arm Rear/hp_out
      mask TypeOptions hp_upr_cg: Upright/hp_upr_cg
      mask TypeOptions hp_upr_wc: Upright/hp_upr_wc
      mask TypeOptions hp_in_rod: Track Rod/hp_in
      mask TypeOptions hp_upr_rod: Track Rod/hp_out | Upright/hp_upr_rod
      mask TypeOptions hp_spr_top: Hardpoints/hp_spr_top | Shock Absorber/hp_spr_top
      mask TypeOptions hp_spr_bot: Shock Absorber/hp_spr_bot | Lower Arm Front/hp_spr
      mask TypeOptions clr_hp: Hardpoints/clr_hp
      mask TypeOptions opc_hp: Hardpoints/opc_hp
      mask TypeOptions size_hp: Hardpoints/size_hp
      mask TypeOptions ua_mass: Upper Arm/ua_mass
      mask TypeOptions clr_ua: Upper Arm/clr_ua
      mask TypeOptions opc_ua: Upper Arm/opc_ua
      mask TypeOptions radius_ua: Upper Arm/radius_ua
      mask TypeOptions laf_mass: Lower Arm Front/rod_mass
      mask TypeOptions lar_mass: Lower Arm Rear/rod_mass
      mask TypeOptions clr_conn_la: Lower Arm Rear/clr_conn_rod | Lower Arm Front/clr_conn_rod
      mask TypeOptions opc_conn_la: Lower Arm Rear/opc_conn_rod | Lower Arm Front/opc_conn_rod
      mask TypeOptions size_conn_la: Lower Arm Rear/size_conn_rod | Lower Arm Front/size_conn_rod
      mask TypeOptions clr_laf: Lower Arm Front/clr_rod
      mask TypeOptions opc_laf: Lower Arm Front/opc_rod
      mask TypeOptions radius_laf: Lower Arm Front/radius_rod
      mask TypeOptions clr_lar: Lower Arm Rear/clr_rod
      mask TypeOptions opc_lar: Lower Arm Rear/opc_rod
      mask TypeOptions radius_lar: Lower Arm Rear/radius_rod
      mask TypeOptions shock_pist_mass: Shock Absorber/shock_pist_mass
      mask TypeOptions shock_cyl_mass: Shock Absorber/shock_cyl_mass
      mask TypeOptions up_lim_bumpstop: Shock Absorber/up_lim_bumpstop
      mask TypeOptions low_lim_bumpstop: Shock Absorber/low_lim_bumpstop
      mask TypeOptions clr_conn_shock: Shock Absorber/clr_conn_shock
      mask TypeOptions opc_conn_shock: Shock Absorber/opc_conn_shock
      mask TypeOptions size_conn_shock: Shock Absorber/size_conn_shock
      mask TypeOptions clr_shock_cyl: Shock Absorber/clr_shock_cyl
      mask TypeOptions opc_shock_cyl: Shock Absorber/opc_shock_cyl
      mask TypeOptions radius_shock_cyl: Shock Absorber/radius_shock_cyl
      mask TypeOptions clr_shock_piston: Shock Absorber/clr_shock_piston
      mask TypeOptions opc_shock_piston: Shock Absorber/opc_shock_piston
      mask TypeOptions clr_shock_bumpstop: Shock Absorber/clr_shock_bumpstop
      mask TypeOptions opc_shock_bumpstop: Shock Absorber/opc_shock_bumpstop
      mask TypeOptions deadvol_len_shock_cyl: Shock Absorber/deadvol_len_shock_cyl
      mask TypeOptions piston_len_shock: Shock Absorber/piston_len_shock
      mask TypeOptions cyl_cap_len_shock: Shock Absorber/cyl_cap_len_shock
      mask TypeOptions bumpstop_len_shock: Shock Absorber/bumpstop_len_shock
      mask TypeOptions atoe: Upright/atoe
      mask TypeOptions acamber: Upright/acamber
      mask TypeOptions upr_mass: Upright/upr_mass
      mask TypeOptions clr_conn_upr: Upright/clr_conn_upr
      mask TypeOptions opc_conn_upr: Upright/opc_conn_upr
      mask TypeOptions size_conn_upr: Upright/size_conn_upr
      mask TypeOptions clr_upr: Upright/clr_upr
      mask TypeOptions opc_upr: Upright/opc_upr
      mask TypeOptions radius_upr: Upright/radius_upr
      mask TypeOptions clr_stub_axle: Upright/clr_stub_axle
      mask TypeOptions opc_stub_axle: Upright/opc_stub_axle
      mask TypeOptions radius_stub_axle: Upright/radius_stub_axle
      mask TypeOptions rod_mass: Track Rod/rod_mass
      mask TypeOptions clr_conn_rod: Track Rod/clr_conn_rod
      mask TypeOptions opc_conn_rod: Track Rod/opc_conn_rod
      mask TypeOptions size_conn_rod: Track Rod/size_conn_rod
      mask TypeOptions clr_rod: Track Rod/clr_rod
      mask TypeOptions opc_rod: Track Rod/opc_rod
      mask TypeOptions radius_rod: Track Rod/radius_rod
      mask DialogControl cont_hp Prompt: Hardpoints
      mask DialogControl cont_vis_hp Prompt: Visualization
      mask DialogControl text_clr_hp Prompt: Color [RGB]
      mask DialogControl text_opc_hp Prompt: Opac. (0-1)
      mask DialogControl text_size_hp Prompt: Size (m)
      mask DialogControl text_hp Prompt: Hardpoints
      mask DialogControl cont_ua Prompt: UA
      mask DialogControl cont_vis_ua Prompt: Visualization
      mask DialogControl cont_laf Prompt: LA
      mask DialogControl text_la_part Prompt: Part
      mask DialogControl text_la_mass Prompt: Mass (kg)
      mask DialogControl text_la_front Prompt: Lower, Front
      mask DialogControl text_la_rear Prompt: Lower, Rear
      mask DialogControl cont_vis_laf Prompt: Visualization
      mask DialogControl text_vis_la_clr Prompt: Color [RGB]
      mask DialogControl text_vis_la_opc Prompt: Opacity (0-1)
      mask DialogControl text_vis_la_rad Prompt: Radius (m)
      mask DialogControl text_vis_la_hp Prompt: Hardpoints
      mask DialogControl text_vis_la_f Prompt: Lower, Front
      mask DialogControl text_vis_la_r Prompt: Lower, Rear
      mask DialogControl cont_shock Prompt: Shock
      mask DialogControl cont_parts Prompt: Parts
      mask DialogControl cont_bumpstop Prompt: Bumpstop
      mask DialogControl cont_vis_shock Prompt: Visualization
      mask DialogControl text_clr_shock Prompt: Color  [RGB]
      mask DialogControl text_opc_shock Prompt: Opac. (0-1)
      mask DialogControl text_size_shock Prompt: Size (m)
      mask DialogControl text_conn_shock Prompt: Connections
      mask DialogControl text_shock_shock Prompt: Cylinder
      mask DialogControl text_shock_piston Prompt: Piston
      mask DialogControl text_piston_radius Prompt: <cylinder radius>
      mask DialogControl text_shock_bumpstop Prompt: Bumpstop
      mask DialogControl text_bumpstop_radius Prompt: <cylinder radius>
      mask DialogControl cont_upright Prompt: Upright
      mask DialogControl grp_upright Prompt: Upright
      mask DialogControl cont_vis_upr Prompt: Visualization
      mask DialogControl text_clr_upr Prompt: Color [RGB]
      mask DialogControl text_opc_upr Prompt: Opac. (0-1)
      mask DialogControl text_size_upr Prompt: Size (m)
      mask DialogControl text_conn_upr Prompt: Connections
      mask DialogControl text_upright Prompt: Upright
      mask DialogControl text_stub_axle Prompt: Stub Axle
      mask DialogControl cont_steer Prompt: Steer
      mask DialogControl grp_rod Prompt: Rod
      mask DialogControl cont_vis_rod Prompt: Visualization
      mask DialogControl text_clr_rod Prompt: Color [RGB]
      mask DialogControl text_opc_rod Prompt: Opac. (0-1)
      mask DialogControl text_size_rod Prompt: Size (m)
      mask DialogControl text_conn_rod Prompt: Connections
      mask DialogControl text_rod_rod Prompt: Rod
      mask DialogControl cont_initial Prompt: Initial
      mask Display: image(fullfile(matlabroot,'toolbox','physmod','sm','smdemos','car_4post_testrig','images','sm_car_4post_dwbR_IMAGE.png'));
  Rack : PMIOPort  Side=Right
  Ref : PMIOPort  Port=2  Side=Right
  Axle : PMIOPort  Port=3  Side=Left
  Brk : PMIOPort  Port=4  Side=Left
  S : PMIOPort  Port=5  Side=Left
  D : PMIOPort  Port=6  Side=Left

== system sm_car_4post_lib/Pulse Input ==
  Gain : Gain  Gain=wave_amplitude
  Ramp : simulink/Sources/Ramp  slope=1/rise_time  start=wave_delay  InitialOutput=0
  Ramp1 : simulink/Sources/Ramp  slope=-1/rise_time  start=wave_delay+pulse_length-rise_time  InitialOutput=0
  Saturation : Saturate  UpperLimit=1  LowerLimit=0
  Saturation1 : Saturate  UpperLimit=0  LowerLimit=-1
  Smooth Step : Subsystem  mask(Smooth step function){step_start=0, step_finish=1, min_out=0, max_out=1}
      mask prompts: step_start "Start Step (u)"; step_finish "Finish Step (u)"; min_out "Minimum output (y)"; max_out "Maximum output (y)"
      mask help:
      | Smooth step function
      | y=3u^2-2u^3
      | Input and output ranges scaled by parameters.
  Sum : Sum  Inputs=|++
  Out1 : Outport  VectorParamsAs1DForOutWhenUnconnected=off
  wires:
  Gain/1 -> Out1/1
  Ramp/1 -> Saturation/1
  Smooth Step/1(y) -> Gain/1
  Saturation/1 -> Sum/1
  Ramp1/1 -> Saturation1/1
  Saturation1/1 -> Sum/2
  Sum/1 -> Smooth Step/1(u)

== system sm_car_4post_lib/Shaft ==
  Shaft : sm_lib/Body Elements/Cylindrical Solid  GraphicAmbientColor=[0.15 0.15 0.15 1.0]  BasedOnType=Mass  CenterOfMass=[0 0 0]  CenterOfMassUnits=m  GraphicDiffuseColor=clr_shaft  CylinderLength=len_shaft  CylinderLengthUnits=m  CylinderRadius=rad_shaft  CylinderRadiusUnits=m  Density=1000  DensityUnits=kg/m^3  DoExposeReferenceFrame=on  GraphicEmissiveColor=[0.0 0.0 0.0 1.0]  ExportEntireGeometry=off  SerializedFrames=<Frames/>  MarkerShape=Sphere  MarkerSize=10  GraphicType=FromGeometry  InertiaType=CalculateFromGeometry  Mass=shaft_m  MassUnits=kg  MomentsOfInertia=[1 1 1]  MomentsOfInertiaUnits=kg*m^2  GraphicOpacity=opc_shaft  ProductsOfInertia=[0 0 0]  ProductsOfInertiaUnits=kg*m^2  GraphicShininess=75  GraphicSpecularColor=[0.5 0.5 0.5 1.0]  GraphicVisPropType=SimpleVisualProperties
  Transform Center : sm_lib/Frames and Transforms/Rigid Transform  TranslationMethod=StandardAxis  TranslationStandardOffset=len_shaft/2*rhs_shaft  TranslationLengthUnit=m  TranslationStandardAxis=-Z  TranslationCartesianOffset=[0 0 0]  TranslationROffset=0  TranslationROffsetUnits=m  TranslationZOffset=0  TranslationZOffsetUnits=m  TranslationThetaOffset=0  TranslationThetaOffsetUnits=deg  RotationMethod=None  RotationAngleUnits=deg  RotationStandardAxis=+Y  RotationAngle=0  RotationArbitraryAxis=[0 0 1]  FollAlignAxisA=+X  BaseAlignAxisA=+Y  FollAlignAxisB=+Y  BaseAlignAxisB=+Z  RotationSequenceAxes=FollowerAxes  RotationSequence=XYX  RotationSequenceAngles=[0 0 0]  RotationSequenceAnglesUnits=deg  RotationMatrix=[1 0 0; 0 1 0; 0 0 1]
  Transform End : sm_lib/Frames and Transforms/Rigid Transform  TranslationMethod=StandardAxis  TranslationStandardOffset=len_shaft/2*rhs_shaft  TranslationLengthUnit=m  TranslationStandardAxis=-Z  TranslationCartesianOffset=[0 0 0]  TranslationROffset=0  TranslationROffsetUnits=m  TranslationZOffset=0  TranslationZOffsetUnits=m  TranslationThetaOffset=0  TranslationThetaOffsetUnits=deg  RotationMethod=None  RotationAngleUnits=deg  RotationStandardAxis=+Y  RotationAngle=0  RotationArbitraryAxis=[0 0 1]  FollAlignAxisA=+X  BaseAlignAxisA=+Y  FollAlignAxisB=+Y  BaseAlignAxisB=+Z  RotationSequenceAxes=FollowerAxes  RotationSequence=XYX  RotationSequenceAngles=[0 0 0]  RotationSequenceAnglesUnits=deg  RotationMatrix=[1 0 0; 0 1 0; 0 0 1]
  B : PMIOPort  Side=Left
  F : PMIOPort  Port=2  Side=Right
  connections:
  Transform End/LConn1 -- Transform Center/RConn1 -- Shaft/RConn1
  Transform Center/LConn1 -- B/RConn1
  F/RConn1 -- Transform End/RConn1
